simulink library "StateVar"  (R2022b)
settings: Solver=VariableStepAuto  StartTime=0.0  StopTime=10.0  RelTol=1e-3
undefined symbols (not defined in the file or in its folder): activeStatePath, MessagePath, ModelRootName, States, Trigger, trigger, TSPs
libraries: $bdroot x3, TSP x1
settings Model: MAModelExclusionFileProxy=C:\work\talariaDev\module\talaria_check_exclusions.xml  Creator=kl13806  LastModifiedBy=kl13806
settings SolverCC: AlgebraicLoopSolver=TrustRegion
settings DebuggingCC: UnconnectedInputMsg=warning  UnconnectedOutputMsg=warning  UnconnectedLineMsg=warning  SFMachineParentedDataDiag=warning  ArithmeticOperatorsInVariantConditions=warning
settings ModelReferenceCC: EnableRefExpFcnMdlSchedulingChecks=on
settings SFSimCC: SimUseLocalCustomCode=off  CustomCodeUndefinedFunction=UseInterfaceOnly
settings RTWCC: RTWUseLocalCustomCode=off  DLArmComputeVersion=19.05
settings CodeAppCC: StateflowObjectComments=on

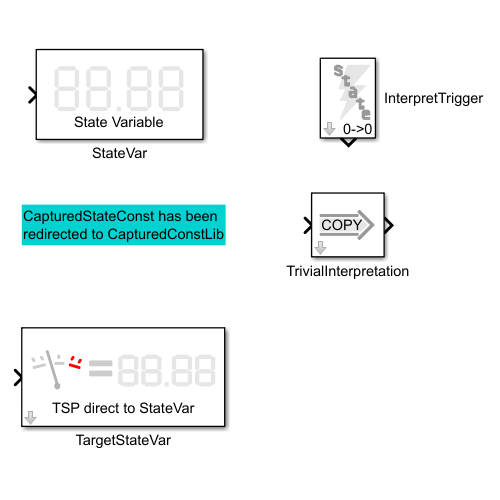
[thumbnail: Simulink's stored preview of the top-level diagram]
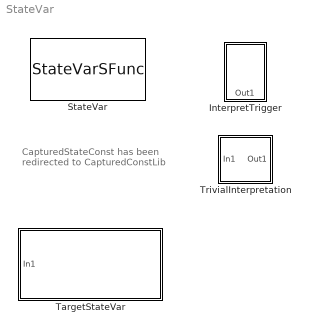
== system StateVar ==
  note: CapturedStateConst has been
      | redirected to CapturedConstLib
  InterpretTrigger : Subsystem  mask(Talaria Interpret Trigger){TriggerInit=[]}
      mask prompts: TriggerInit "Hidden: MoveFcn redraw"
      mask help: This block generates a function trigger to drive interpretation blocks
      mask init:
      | [ok,Trigger,States,TSPs] = InterpretTriggerMask.Init(gcbh);
      settings: MoveFcn=InterpretTriggerMask.CB_TriggerInit(gcbh);
      mask Callback TriggerInit: InterpretTriggerMask.CB_TriggerInit(gcbh);
      mask DialogControl ButtonCreateInterpretation Prompt: Create sample interpretation blocks
      mask DialogControl ButtonCreateInterpretation Callback: InterpretTriggerMask.CreateEmptyInterpretation(gcbh);
      mask DialogControl ButtonResizeInterpreter Prompt: Auto-size interpreter block
      mask DialogControl ButtonResizeInterpreter Callback: InterpretTriggerMask.CB_ResizeInterpreter(gcbh);
      mask DialogControl ButtonEditData Prompt: Launch "Edit Data" dialog
      mask DialogControl ButtonEditData Callback: InterpretTriggerMask.CB_EditData(gcbh);
      mask DialogControl ButtonEditScript Prompt: Edit script
      mask DialogControl ButtonEditScript Callback: InterpretTriggerMask.CB_EditScript(gcbh);
      mask DialogControl ButtonAutoName Prompt: Rename script In and Out arguments based on blocks
      mask DialogControl ButtonAutoName Callback: InterpretTriggerMask.CB_AutoNameArguments(gcbh);
      mask DialogControl ButtonRunInterpretation Prompt:
      | Attempt to run interpretation right now
      | (Experimental. Ensure successful simulation or data load first)
      mask DialogControl ButtonRunInterpretation Callback: InterpretTriggerMask.CB_RunInterpretation(gcbh);
      mask DialogControl ErrorContainer Prompt: Error Messages
      mask Display:
      | % retrieve icon definition
      | [path,w,h] = InterpretTriggerMask.Icon();
      | 
      | % retrieve the block's pixel size
      | pos = get(gcbh,'position');
      | bw = pos(3) - pos(1);
      | bh = pos(4) - pos(2);
      | 
      | % draw centered icon
      | xAdj = bw/2 - w/2 + 3;
      | yAdj = bh/2 - h/2 + 4;
      | for i=1:length(path)
      |    %path(i).x(end+1) = path(i).x(1);
      |    %path(i).y(end+1) = path(i).y(1);
      |    %plot(path(i).x+xAdj, path(i).y+yAdj);
      |    patch(path(i).x+xAdj, path(i).y+yAdj, path(i).rgb);
      | end
      | 
      | % display a count of how many dependent TSPs we found
      | outCount = 0;
      | inCount = 0;
      | if (exist('TSPs') && ~isempty(TSPs))
      |     inCount = length(strfind(TSPs,',')) + 1;
      | end
      | if (exist('States') && ~isempty(States))
      |     outCount = length(strfind(States,',')) + 1;
      | end
      | inoutTxt = sprintf('%d->%d',inCount,outCount);
      | text(bw-2, 0, inoutTxt, 'horizontalAlignment', 'right', ...
      |      'verticalAlignment', 'bottom');
      | 
      | % show the name or an X
      | if (exist('ok','var') && ok)
      | 	%text(bw*0.5, bh*0.15, 'Interpret', 'horizontalAlignment','center');
      | 	patch(0,0,[1 1 1]);
      | 	patch(bw,bh,[1 1 1]);
      | else
      | 	tx=bw*0.03;
      | 	ty=bh*0.03;
      | 	patch([0 tx bw bw-tx], [ty 0 bh-ty bh], [1 0 0]);
      | 	patch([0 bw-tx bw tx], [bh-ty 0 ty bh], [1 0 0]);
      | end
  StateVar : M-S-Function  FunctionName=StateVarSFunc  Parameters=activeStatePath,trigger  mask(Talaria State Variable){TriggerInit=[85 19 200 81], StateName=}
      mask prompts: TriggerInit "Hidden: MoveFcn redraw"; StateName "Name:"
      mask help: The State Variable (StateVar) block receives the interpreted target state data as part of the State Interpretation Engine.
      mask init:
      | [ok,activeStatePath,trigger] = StateVarMask.Init(gcbh,StateName);
      settings: MoveFcn=StateVarMask.CB_TriggerInit(gcbh);
      mask Callback TriggerInit: StateVarMask.CB_TriggerInit(gcbh);
      mask DialogControl ValuePrompt Prompt: Value:
      mask DialogControl ValueText Prompt: double([])
      mask DialogControl ButtonEditValue Prompt: Directly Edit Value
      mask DialogControl ButtonEditValue Callback: DataMapHelper.CB_EditDialog(gcbh,StateVarMask.DataMap,'Value');
      mask DialogControl ErrorContainer Prompt: Error Messages
      mask Display:
      | % retrieve icon definition
      | [path,w,h] = StateVarMask.Icon();
      | 
      | % retrieve the block's pixel size
      | pos = get(gcbh,'position');
      | bw = pos(3) - pos(1);
      | bh = pos(4) - pos(2);
      | 
      | % draw centered icon
      | xAdj = bw/2 - w/2;
      | yAdj = bh/2 - h/2 + 4;
      | for i=1:length(path)
      | 	patch(path(i).x+xAdj, path(i).y+yAdj, path(i).rgb);
      | end
      | 
      | % show the state name or an X
      | if (exist('ok','var') && ok)
      | 	text(bw*0.5, bh*0.2, activeStatePath, 'horizontalAlignment', 'center');
      | 	patch(0,0,[1 1 1]);
      | 	patch(bw,bh,[1 1 1]);
      | else
      | 	tx=bw*0.03;
      | 	ty=bh*0.03;
      | 	patch([0 tx bw bw-tx], [ty 0 bh-ty bh], [1 0 0]);
      | 	patch([0 bw-tx bw tx], [bh-ty 0 ty bh], [1 0 0]);
      | end
  TargetStateVar : Subsystem  mask(Talaria Target State Variable){TriggerInit=[75 211 215 279], TspName=, StateName=, UseSameName=on, IfdefMacro=[]}
      mask prompts: TriggerInit "Hidden: MoveFcn redraw"; TspName "Name:"; StateName "Name of StateVar:"; UseSameName "Use same name for state variable and TSP"; IfdefMacro "Additional #ifdef macro to enable trigger capture:"
      mask help: The TargetStateVar block encapsultes a Target State Probe (TSP), a State Variable, and a Trivial Interpretation between them.
      mask init:
      | [ok,tspPath,activeStatePath] = TargetStateVarMask.Init(gcbh);
      settings: MoveFcn=TargetStateVarMask.CB_TriggerInit(gcbh);
      mask Help: See help for StateVar and TSP blocks
      mask Callback TriggerInit: TargetStateVarMask.CB_TriggerInit(gcbh);
      mask TypeOptions TspName: TSP/TspName
      mask TypeOptions StateName: StateVar/StateName
      mask Callback UseSameName: TargetStateVarMask.CB_UseSameName(gcbh);
      mask TypeOptions IfdefMacro: TSP/IfdefMacro
      mask DialogControl AdvancedPanel Prompt: Advanced
      mask DialogControl ConvertToFullInterpretation Prompt: Irreversible conversion to full interpretation
      mask DialogControl ConvertToFullInterpretation Callback: TargetStateVarMask.CB_ConvertToFullInterpretation(gcbh);
      mask DialogControl ErrorContainer Prompt: Error Messages
      mask Display:
      | % retrieve icon definition
      | [path,w,h] = TargetStateVarMask.Icon();
      | 
      | % retrieve the block's pixel size
      | pos = get(gcbh,'position');
      | bw = pos(3) - pos(1);
      | bh = pos(4) - pos(2);
      | 
      | % draw centered icon
      | xAdj = bw/2 - w/2 + 5;
      | yAdj = bh/2 - h/2 + 4;
      | for i=1:length(path)
      | 	patch(path(i).x+xAdj, path(i).y+yAdj, path(i).rgb);
      | end
      | 
      | % show the top name or an X
      | if (exist('ok','var') && ok)
      | 	text(bw*0.5, bh*0.2, tspPath, 'horizontalAlignment', 'center');
      | 	patch(0,0,[1 1 1]);
      | 	patch(bw,bh,[1 1 1]);
      | else
      | 	tx=bw*0.03;
      | 	ty=bh*0.03;
      | 	patch([0 tx bw bw-tx], [ty 0 bh-ty bh], [1 0 0]);
      | 	patch([0 bw-tx bw tx], [bh-ty 0 ty bh], [1 0 0]);
      | end
  TrivialInterpretation : Subsystem  mask(Talaria Trivial Interpretation){TriggerInit=[]}
      mask prompts: TriggerInit "Hidden: MoveFcn redraw"
      mask help: A trivial interpreter connects to a TSP on the input side and to a StateVar for output. The interpreter then simply copies the value from TSP to StateVar with no changes.
      mask init:
      | TrivialInterpretationMask.Init(gcbh);
      settings: MoveFcn=TrivialInterpretationMask.CB_TriggerInit(gcbh);
      mask Callback TriggerInit: TrivialInterpretationMask.CB_TriggerInit(gcbh);
      mask Display:
      | % retrieve icon definition
      | [path,w,h] = TrivialInterpretationMask.Icon();
      | 
      | % retrieve the block's pixel size
      | pos = get(gcbh,'position');
      | bw = pos(3) - pos(1);
      | bh = pos(4) - pos(2);
      | 
      | % draw centered icon
      | xAdj = bw/2 - w/2;
      | yAdj = bh/2 - h/2;
      | for i=1:length(path)
      |    patch(path(i).x+xAdj, path(i).y+yAdj, path(i).rgb);
      | end
      | disp('COPY   ');

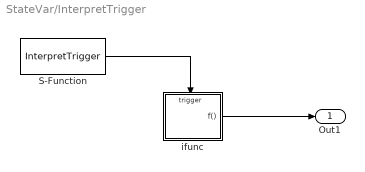
== system StateVar/InterpretTrigger ==
  S-Function : S-Function  FunctionName=InterpretTrigger  Parameters=Trigger,TSPs,States,0  SFunctionDeploymentMode=off  EnableBusSupport=off
  ifunc : MATLAB Function  TreatAsAtomicUnit=on  RTWFcnName=['RtcReqRsp_' MessagePath]  RTWFileName=[ModelRootName(bdroot) '_RTC_REQ_RSP']
      settings: RTWSystemCode=Nonreusable function
  Out1 : Outport  VectorParamsAs1DForOutWhenUnconnected=off
  wires:
  S-Function/1 -> ifunc/Trigger
  ifunc/1(f()) -> Out1/1

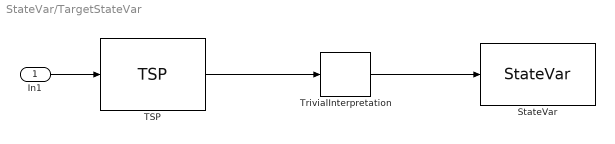
== system StateVar/TargetStateVar ==
  In1 : Inport
  StateVar : $bdroot/StateVar  TriggerInit=[490 139 605 201]
  TSP : TSP/TSP  TriggerInit=[110 134 215 206]  IfDefMacro=IfdefMacro  Role=Automatic
      settings: SourceProductName=Bose Talaria
  TrivialInterpretation : $bdroot/TrivialInterpretation  TriggerInit=[330 148 380 192]
  wires:
  TSP/1 -> TrivialInterpretation/1
  TrivialInterpretation/1 -> StateVar/1
  In1/1 -> TSP/1

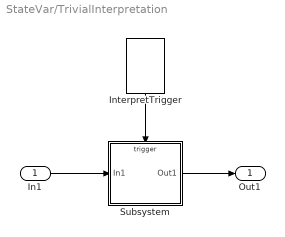
== system StateVar/TrivialInterpretation ==
  In1 : Inport
  InterpretTrigger : $bdroot/InterpretTrigger  TriggerInit=[266 15 304 70]
  Subsystem : Subsystem
  Out1 : Outport  VectorParamsAs1DForOutWhenUnconnected=off
  wires:
  In1/1 -> Subsystem/1(In1)
  InterpretTrigger/1 -> Subsystem/Trigger
  Subsystem/1(Out1) -> Out1/1

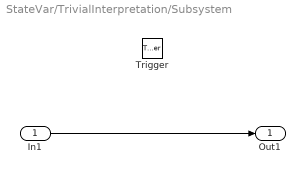
== system StateVar/TrivialInterpretation/Subsystem ==
  In1 : Inport
  Trigger : TriggerPort  TriggerType=function-call  VariantControl=Variant  PortDimensions=1
  Out1 : Outport  VectorParamsAs1DForOutWhenUnconnected=off
  wires:
  In1/1 -> Out1/1

== matlab function StateVar/InterpretTrigger/ifunc ==
  events: trigger input FUNCTION_CALL_EVENT; f output FUNCTION_CALL_EVENT
function fcn
% This function serves only to invoke a function trigger output
f();
